simulink model "aircraft_fixd"  (R2016a)
settings: Solver=ode45  StartTime=0.0  StopTime=1000  RelTol=1e-3
undefined symbols (not defined in the file): Newton, Raphson
libraries: simulink x7, aerolibasang x5, aerolib6dof2 x1
settings Model: Creator=HELLO  LastModifiedBy=lsr
settings DataIOCC: LimitDataPoints=on  SaveFormat=Array
settings DebuggingCC: SolverPrmCheckMsg=warning
settings HardwareCC: ProdBitPerPointer=32  ProdLargestAtomicFloat=None  ProdIntDivRoundTo=Undefined  ProdEndianess=Unspecified  ProdWordSize=32  ProdHWDeviceType=32-bit Generic
settings ModelReferenceCC: PropagateSignalLabelsOutOfModel=off
settings ConfigComp: CovModelRefEnable=Off  CovSFcnEnable=off

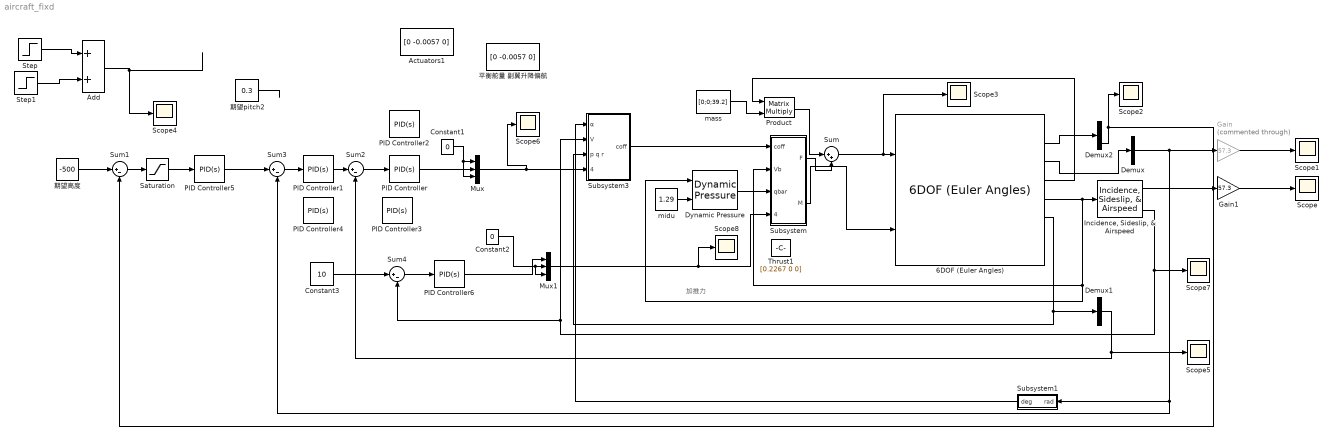
== system aircraft_fixd ==
  note: 加推力
  6DOF (Euler Angles) : aerolib6dof2/6DOF (Euler Angles)  units=Metric (MKS)  mtype=Fixed  rep=Euler Angles  xme_0=[100 0 -200]  Vm_0=[15 0 0]  eul_0=[0 0 0]  pm_0=[0 0 0]  mass_0=4  mass_e=0.5  mass_f=2.0  inertia=[0.1 0 0;0 0.05 0;0 0 0.1]  inertia_e=eye(3)  inertia_f=2*eye(3)  k_quat=1.0  vre_flag=on
  Actuators1 : Constant  Value=[0 -0.0057 0]
  Add : Sum
  Constant1 : Constant  Value=0
  Constant2 : Constant  Value=0
  Constant3 : Constant  Value=10
  Demux : Demux  Outputs=3
  Demux1 : Demux  Outputs=3
  Demux2 : Demux  Outputs=3
  Dynamic Pressure : aerolibasang/Dynamic Pressure
  Gain : Gain  Commented=through  Gain=57.3
  Gain1 : Gain  Gain=57.3
  "Incidence, Sideslip, & Airspeed" : aerolibasang/Incidence, Sideslip, & Airspeed
  Mux : Mux  Inputs=3
  Mux1 : Mux  Inputs=3
  PID Controller : simulink/Continuous/PID Controller  Controller=PID  TimeDomain=Continuous-time  SampleTime=-1  IntegratorMethod=Forward Euler  FilterMethod=Forward Euler  Form=Parallel  UseFilter=on  ControllerParametersSource=internal  P=-0.5  I=-0.01  D=0  N=100  InitialConditionSource=internal  InitialConditionForIntegrator=0  InitialConditionForFilter=0  ExternalReset=none  LimitOutput=off  UpperSaturationLimit=inf  LowerSaturationLimit=-inf  LinearizeAsGain=on  AntiWindupMode=none  Kb=1  TrackingMode=off  Kt=1  PParamMin=[]  PParamMax=[]  IParamMin=[]  IParamMax=[]  DParamMin=[]  DParamMax=[]  NParamMin=[]  NParamMax=[]  KbParamMin=[]  KbParamMax=[]  KtParamMin=[]  KtParamMax=[]  POutMin=[]  POutMax=[]  IOutMin=[]  IOutMax=[]  DOutMin=[]  DOutMax=[]  NOutMin=[]  NOutMax=[]  KbOutMin=[]  KbOutMax=[]  KtOutMin=[]  KtOutMax=[]  IntegratorOutMin=[]  IntegratorOutMax=[]  FilterOutMin=[]  FilterOutMax=[]  SumOutMin=[]  SumOutMax=[]  SumI1OutMin=[]  SumI1OutMax=[]  SumI2OutMin=[]  SumI2OutMax=[]  SumI3OutMin=[]  SumI3OutMax=[]  SumDOutMin=[]  SumDOutMax=[]  SaturationOutMin=[]  SaturationOutMax=[]  IntegratorContinuousStateAttributes=''  IntegratorStateMustResolveToSignalObject=off  IntegratorRTWStateStorageClass=Auto  FilterContinuousStateAttributes=''  FilterStateMustResolveToSignalObject=off  FilterRTWStateStorageClass=Auto  DifferentiatorICPrevScaledInput=0  DifferentiatorOutMin=[]  DifferentiatorOutMax=[]
  PID Controller1 : simulink/Continuous/PID Controller  Controller=PID  TimeDomain=Continuous-time  SampleTime=-1  IntegratorMethod=Forward Euler  FilterMethod=Forward Euler  Form=Parallel  UseFilter=on  ControllerParametersSource=internal  P=0.1  I=0.3  D=0.1  N=100  InitialConditionSource=internal  InitialConditionForIntegrator=0  InitialConditionForFilter=0  ExternalReset=none  LimitOutput=off  UpperSaturationLimit=inf  LowerSaturationLimit=-inf  LinearizeAsGain=on  AntiWindupMode=none  Kb=1  TrackingMode=off  Kt=1  PParamMin=[]  PParamMax=[]  IParamMin=[]  IParamMax=[]  DParamMin=[]  DParamMax=[]  NParamMin=[]  NParamMax=[]  KbParamMin=[]  KbParamMax=[]  KtParamMin=[]  KtParamMax=[]  POutMin=[]  POutMax=[]  IOutMin=[]  IOutMax=[]  DOutMin=[]  DOutMax=[]  NOutMin=[]  NOutMax=[]  KbOutMin=[]  KbOutMax=[]  KtOutMin=[]  KtOutMax=[]  IntegratorOutMin=[]  IntegratorOutMax=[]  FilterOutMin=[]  FilterOutMax=[]  SumOutMin=[]  SumOutMax=[]  SumI1OutMin=[]  SumI1OutMax=[]  SumI2OutMin=[]  SumI2OutMax=[]  SumI3OutMin=[]  SumI3OutMax=[]  SumDOutMin=[]  SumDOutMax=[]  SaturationOutMin=[]  SaturationOutMax=[]  IntegratorContinuousStateAttributes=''  IntegratorStateMustResolveToSignalObject=off  IntegratorRTWStateStorageClass=Auto  FilterContinuousStateAttributes=''  FilterStateMustResolveToSignalObject=off  FilterRTWStateStorageClass=Auto  DifferentiatorICPrevScaledInput=0  DifferentiatorOutMin=[]  DifferentiatorOutMax=[]
  PID Controller2 : simulink/Continuous/PID Controller  Controller=PID  TimeDomain=Continuous-time  SampleTime=-1  IntegratorMethod=Forward Euler  FilterMethod=Forward Euler  Form=Parallel  UseFilter=on  ControllerParametersSource=internal  P=-0.6  I=-0.01  D=0  N=100  InitialConditionSource=internal  InitialConditionForIntegrator=0  InitialConditionForFilter=0  ExternalReset=none  LimitOutput=off  UpperSaturationLimit=inf  LowerSaturationLimit=-inf  LinearizeAsGain=on  AntiWindupMode=none  Kb=1  TrackingMode=off  Kt=1  PParamMin=[]  PParamMax=[]  IParamMin=[]  IParamMax=[]  DParamMin=[]  DParamMax=[]  NParamMin=[]  NParamMax=[]  KbParamMin=[]  KbParamMax=[]  KtParamMin=[]  KtParamMax=[]  POutMin=[]  POutMax=[]  IOutMin=[]  IOutMax=[]  DOutMin=[]  DOutMax=[]  NOutMin=[]  NOutMax=[]  KbOutMin=[]  KbOutMax=[]  KtOutMin=[]  KtOutMax=[]  IntegratorOutMin=[]  IntegratorOutMax=[]  FilterOutMin=[]  FilterOutMax=[]  SumOutMin=[]  SumOutMax=[]  SumI1OutMin=[]  SumI1OutMax=[]  SumI2OutMin=[]  SumI2OutMax=[]  SumI3OutMin=[]  SumI3OutMax=[]  SumDOutMin=[]  SumDOutMax=[]  SaturationOutMin=[]  SaturationOutMax=[]  IntegratorContinuousStateAttributes=''  IntegratorStateMustResolveToSignalObject=off  IntegratorRTWStateStorageClass=Auto  FilterContinuousStateAttributes=''  FilterStateMustResolveToSignalObject=off  FilterRTWStateStorageClass=Auto  DifferentiatorICPrevScaledInput=0  DifferentiatorOutMin=[]  DifferentiatorOutMax=[]
  PID Controller3 : simulink/Continuous/PID Controller  Controller=PID  TimeDomain=Continuous-time  SampleTime=-1  IntegratorMethod=Forward Euler  FilterMethod=Forward Euler  Form=Parallel  UseFilter=on  ControllerParametersSource=internal  P=-0.3  I=-0.01  D=0  N=100  InitialConditionSource=internal  InitialConditionForIntegrator=0  InitialConditionForFilter=0  ExternalReset=none  LimitOutput=off  UpperSaturationLimit=inf  LowerSaturationLimit=-inf  LinearizeAsGain=on  AntiWindupMode=none  Kb=1  TrackingMode=off  Kt=1  PParamMin=[]  PParamMax=[]  IParamMin=[]  IParamMax=[]  DParamMin=[]  DParamMax=[]  NParamMin=[]  NParamMax=[]  KbParamMin=[]  KbParamMax=[]  KtParamMin=[]  KtParamMax=[]  POutMin=[]  POutMax=[]  IOutMin=[]  IOutMax=[]  DOutMin=[]  DOutMax=[]  NOutMin=[]  NOutMax=[]  KbOutMin=[]  KbOutMax=[]  KtOutMin=[]  KtOutMax=[]  IntegratorOutMin=[]  IntegratorOutMax=[]  FilterOutMin=[]  FilterOutMax=[]  SumOutMin=[]  SumOutMax=[]  SumI1OutMin=[]  SumI1OutMax=[]  SumI2OutMin=[]  SumI2OutMax=[]  SumI3OutMin=[]  SumI3OutMax=[]  SumDOutMin=[]  SumDOutMax=[]  SaturationOutMin=[]  SaturationOutMax=[]  IntegratorContinuousStateAttributes=''  IntegratorStateMustResolveToSignalObject=off  IntegratorRTWStateStorageClass=Auto  FilterContinuousStateAttributes=''  FilterStateMustResolveToSignalObject=off  FilterRTWStateStorageClass=Auto  DifferentiatorICPrevScaledInput=0  DifferentiatorOutMin=[]  DifferentiatorOutMax=[]
  PID Controller4 : simulink/Continuous/PID Controller  Controller=PID  TimeDomain=Continuous-time  SampleTime=-1  IntegratorMethod=Forward Euler  FilterMethod=Forward Euler  Form=Parallel  UseFilter=on  ControllerParametersSource=internal  P=0.1  I=0.25  D=0.1  N=100  InitialConditionSource=internal  InitialConditionForIntegrator=0  InitialConditionForFilter=0  ExternalReset=none  LimitOutput=off  UpperSaturationLimit=inf  LowerSaturationLimit=-inf  LinearizeAsGain=on  AntiWindupMode=none  Kb=1  TrackingMode=off  Kt=1  PParamMin=[]  PParamMax=[]  IParamMin=[]  IParamMax=[]  DParamMin=[]  DParamMax=[]  NParamMin=[]  NParamMax=[]  KbParamMin=[]  KbParamMax=[]  KtParamMin=[]  KtParamMax=[]  POutMin=[]  POutMax=[]  IOutMin=[]  IOutMax=[]  DOutMin=[]  DOutMax=[]  NOutMin=[]  NOutMax=[]  KbOutMin=[]  KbOutMax=[]  KtOutMin=[]  KtOutMax=[]  IntegratorOutMin=[]  IntegratorOutMax=[]  FilterOutMin=[]  FilterOutMax=[]  SumOutMin=[]  SumOutMax=[]  SumI1OutMin=[]  SumI1OutMax=[]  SumI2OutMin=[]  SumI2OutMax=[]  SumI3OutMin=[]  SumI3OutMax=[]  SumDOutMin=[]  SumDOutMax=[]  SaturationOutMin=[]  SaturationOutMax=[]  IntegratorContinuousStateAttributes=''  IntegratorStateMustResolveToSignalObject=off  IntegratorRTWStateStorageClass=Auto  FilterContinuousStateAttributes=''  FilterStateMustResolveToSignalObject=off  FilterRTWStateStorageClass=Auto  DifferentiatorICPrevScaledInput=0  DifferentiatorOutMin=[]  DifferentiatorOutMax=[]
  PID Controller5 : simulink/Continuous/PID Controller  Controller=PID  TimeDomain=Continuous-time  SampleTime=-1  IntegratorMethod=Forward Euler  FilterMethod=Forward Euler  Form=Parallel  UseFilter=on  ControllerParametersSource=internal  P=-0.1  I=0  D=0  N=100  InitialConditionSource=internal  InitialConditionForIntegrator=0  InitialConditionForFilter=0  ExternalReset=none  LimitOutput=off  UpperSaturationLimit=inf  LowerSaturationLimit=-inf  LinearizeAsGain=on  AntiWindupMode=none  Kb=1  TrackingMode=off  Kt=1  PParamMin=[]  PParamMax=[]  IParamMin=[]  IParamMax=[]  DParamMin=[]  DParamMax=[]  NParamMin=[]  NParamMax=[]  KbParamMin=[]  KbParamMax=[]  KtParamMin=[]  KtParamMax=[]  POutMin=[]  POutMax=[]  IOutMin=[]  IOutMax=[]  DOutMin=[]  DOutMax=[]  NOutMin=[]  NOutMax=[]  KbOutMin=[]  KbOutMax=[]  KtOutMin=[]  KtOutMax=[]  IntegratorOutMin=[]  IntegratorOutMax=[]  FilterOutMin=[]  FilterOutMax=[]  SumOutMin=[]  SumOutMax=[]  SumI1OutMin=[]  SumI1OutMax=[]  SumI2OutMin=[]  SumI2OutMax=[]  SumI3OutMin=[]  SumI3OutMax=[]  SumDOutMin=[]  SumDOutMax=[]  SaturationOutMin=[]  SaturationOutMax=[]  IntegratorContinuousStateAttributes=''  IntegratorStateMustResolveToSignalObject=off  IntegratorRTWStateStorageClass=Auto  FilterContinuousStateAttributes=''  FilterStateMustResolveToSignalObject=off  FilterRTWStateStorageClass=Auto  DifferentiatorICPrevScaledInput=0  DifferentiatorOutMin=[]  DifferentiatorOutMax=[]
  PID Controller6 : simulink/Continuous/PID Controller  Controller=PID  TimeDomain=Continuous-time  SampleTime=-1  IntegratorMethod=Forward Euler  FilterMethod=Forward Euler  Form=Parallel  UseFilter=on  ControllerParametersSource=internal  P=2  I=0  D=0  N=100  InitialConditionSource=internal  InitialConditionForIntegrator=0  InitialConditionForFilter=0  ExternalReset=none  LimitOutput=off  UpperSaturationLimit=inf  LowerSaturationLimit=-inf  LinearizeAsGain=on  AntiWindupMode=none  Kb=1  TrackingMode=off  Kt=1  PParamMin=[]  PParamMax=[]  IParamMin=[]  IParamMax=[]  DParamMin=[]  DParamMax=[]  NParamMin=[]  NParamMax=[]  KbParamMin=[]  KbParamMax=[]  KtParamMin=[]  KtParamMax=[]  POutMin=[]  POutMax=[]  IOutMin=[]  IOutMax=[]  DOutMin=[]  DOutMax=[]  NOutMin=[]  NOutMax=[]  KbOutMin=[]  KbOutMax=[]  KtOutMin=[]  KtOutMax=[]  IntegratorOutMin=[]  IntegratorOutMax=[]  FilterOutMin=[]  FilterOutMax=[]  SumOutMin=[]  SumOutMax=[]  SumI1OutMin=[]  SumI1OutMax=[]  SumI2OutMin=[]  SumI2OutMax=[]  SumI3OutMin=[]  SumI3OutMax=[]  SumDOutMin=[]  SumDOutMax=[]  SaturationOutMin=[]  SaturationOutMax=[]  IntegratorContinuousStateAttributes=''  IntegratorStateMustResolveToSignalObject=off  IntegratorRTWStateStorageClass=Auto  FilterContinuousStateAttributes=''  FilterStateMustResolveToSignalObject=off  FilterRTWStateStorageClass=Auto  DifferentiatorICPrevScaledInput=0  DifferentiatorOutMin=[]  DifferentiatorOutMax=[]
  Product : Product  Multiplication=Matrix(*)
  Saturation : Saturate  UpperLimit=10  LowerLimit=-10
  Scope{,1..8} (9 alike) : Scope
  Step : Step  Time=2  After=0.1  SampleTime=0
  Step1 : Step  Time=2.1  After=-0.1  SampleTime=0
  Subsystem : Subsystem
  Subsystem1 : Subsystem
  Subsystem3 : Subsystem
  Sum : Sum  Inputs=|++
  Sum{1..4} (4 alike) : Sum  Inputs=|+-
  Thrust1 : Constant  Value=[0.2267 0 0]
  mass : Constant  Value=[0;0;39.2]
  midu : Constant  Value=1.29
  平衡舵量 副翼升降偏航 : Constant  Value=[0 -0.0057 0]
  期望pitch2 : Constant  Value=0.3
  期望高度 : Constant  Value=-500
  wires:
  Subsystem3/1(coff) -> Subsystem/1(coff)
  Mux1/1 -> Scope8/1, Subsystem/4(Thurst)
  Subsystem/2(M) -> 6DOF (Euler Angles)/2
  6DOF (Euler Angles)/5 -> Subsystem/2(Vb), Dynamic Pressure/1, "Incidence, Sideslip, & Airspeed"/1
  6DOF (Euler Angles)/6 -> Demux1/1, Subsystem3/3(p q r)
  midu/1 -> Dynamic Pressure/2
  Dynamic Pressure/1 -> Subsystem/3(qbar)
  mass/1 -> Product/2
  6DOF (Euler Angles)/4 -> Product/1
  Product/1 -> Sum/1
  Sum/1 -> Scope3/1, 6DOF (Euler Angles)/1
  Subsystem/1(F) -> Sum/2
  "Incidence, Sideslip, & Airspeed"/3 -> Scope7/1, Sum4/2, Subsystem3/2(V)
  6DOF (Euler Angles)/2 -> Demux2/1
  "Incidence, Sideslip, & Airspeed"/1 -> Gain1/1
  Subsystem1/1(deg) -> Subsystem3/1(α)
  6DOF (Euler Angles)/3 -> Demux/1
  Demux/2 -> Subsystem1/1(rad), Sum3/2, Gain/1
  Step/1 -> Add/1
  Step1/1 -> Add/2
  Add/1 -> Scope4/1
  Demux1/2 -> Scope5/1, Sum2/2
  Sum2/1 -> PID Controller/1
  PID Controller1/1 -> Sum2/1
  Mux/1 -> Scope6/1, Subsystem3/4(Actuators)
  PID Controller/1 -> Mux/2
  Constant1/1 -> Mux/3, Mux/1
  Sum3/1 -> PID Controller1/1
  PID Controller5/1 -> Sum3/1
  Gain/1 -> Scope1/1
  Gain1/1 -> Scope/1
  Sum1/1 -> Saturation/1
  期望高度/1 -> Sum1/1
  Demux2/3 -> Sum1/2, Scope2/1
  期望pitch2/1 -> ?
  Saturation/1 -> PID Controller5/1
  Constant2/1 -> Mux1/2, Mux1/3
  PID Controller6/1 -> Mux1/1
  Sum4/1 -> PID Controller6/1
  Constant3/1 -> Sum4/1

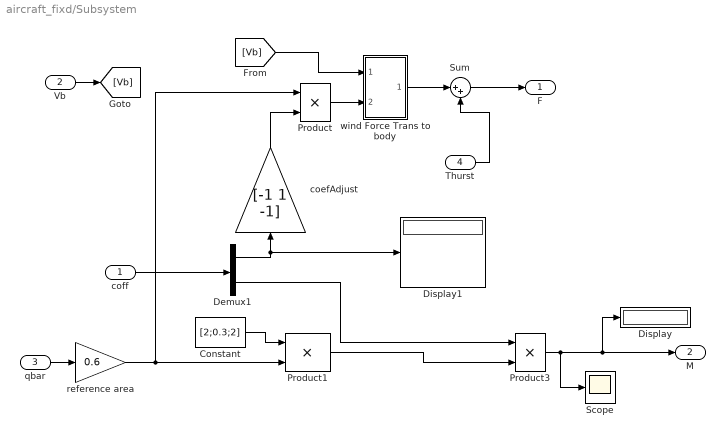
== system aircraft_fixd/Subsystem ==
  coff : Inport
  Vb : Inport  Port=2
  qbar : Inport  Port=3
  Thurst : Inport  Port=4
  Constant : Constant  Value=[2;0.3;2]
  Demux1 : Demux  Outputs=[3,3]
  Display : Display
  Display1 : Display
  Product : Product  SaturateOnIntegerOverflow=on  InputSameDT=on  OutDataTypeStr=Inherit: Same as first input
  Product1 : Product  SaturateOnIntegerOverflow=on  InputSameDT=on  OutDataTypeStr=Inherit: Same as first input
  Product3 : Product  SaturateOnIntegerOverflow=on  InputSameDT=on  OutDataTypeStr=Inherit: Same as first input
  Scope : Scope
  Sum : Sum  Inputs=|++
  coefAdjust : Gain  Gain="[-1  1  -1]"
  reference area : Gain  Gain=0.6  SaturateOnIntegerOverflow=on  OutDataTypeStr=Inherit: Same as input  ParamDataTypeStr=Inherit: Same as input
  wind Force Trans to body : Subsystem
  F : Outport
  M : Outport  Port=2
  wires:
  Product1/1 -> Product3/2
  Constant/1 -> Product1/1
  coff/1 -> Demux1/1
  Demux1/2 -> Product3/1
  qbar/1 -> reference area/1
  reference area/1 -> Product1/2, Product/1
  Demux1/1 -> coefAdjust/1, Display1/1
  Vb/1 -> [Vb]
  coefAdjust/1 -> Product/2
  Thurst/1 -> Sum/2
  Product3/1 -> M/1, Display/1, Scope/1
  Sum/1 -> F/1
  [Vb] -> wind Force Trans to body/1(In1)
  Product/1 -> wind Force Trans to body/2(In2)
  wind Force Trans to body/1(Out1) -> Sum/1

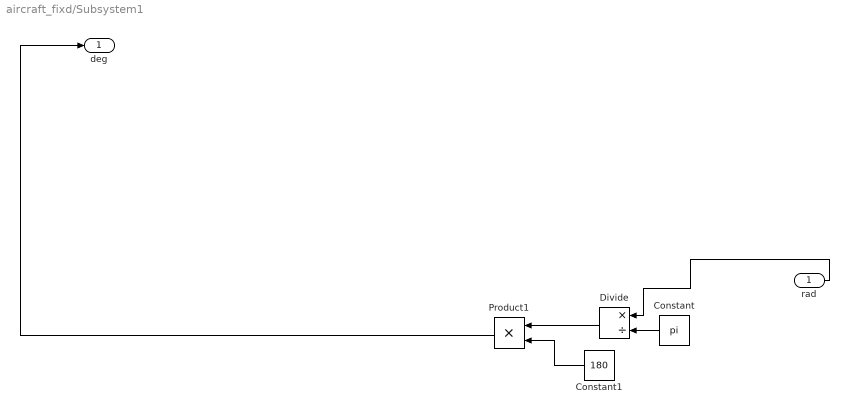
== system aircraft_fixd/Subsystem1 ==
  rad : Inport
  Constant : Constant  Value=pi
  Constant1 : Constant  Value=180
  Divide : Product  Inputs=*/
  Product1 : Product
  deg : Outport
  wires:
  Constant/1 -> Divide/2
  Product1/1 -> deg/1
  Constant1/1 -> Product1/2
  Divide/1 -> Product1/1
  rad/1 -> Divide/1

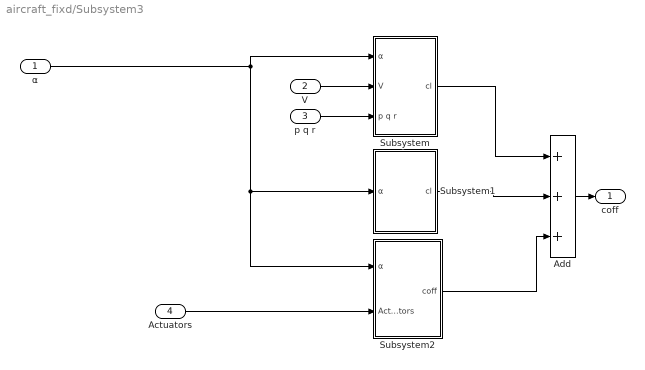
== system aircraft_fixd/Subsystem3 ==
  α : Inport
  V : Inport  Port=2
  p q r : Inport  Port=3
  Actuators : Inport  Port=4
  Add : Sum  Inputs=+++
  Subsystem : Subsystem
  Subsystem1 : Subsystem
  Subsystem2 : Subsystem
  coff : Outport
  wires:
  p q r/1 -> Subsystem/3(p q r)
  V/1 -> Subsystem/2(V)
  Actuators/1 -> Subsystem2/2(Actuators)
  Subsystem1/1(cl) -> Add/2
  Subsystem/1(cl) -> Add/1
  Subsystem2/1(coff) -> Add/3
  Add/1 -> coff/1
  α/1 -> Subsystem/1(α), Subsystem2/1(α), Subsystem1/1(α)

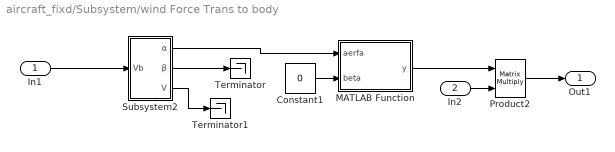
== system aircraft_fixd/Subsystem/wind Force Trans to body ==
  In1 : Inport
  In2 : Inport  Port=2
  Constant1 : Constant  Value=0
  MATLAB Function : MATLAB Function  TreatAsAtomicUnit=on
  Product2 : Product  Multiplication=Matrix(*)  SaturateOnIntegerOverflow=on  InputSameDT=on  OutDataTypeStr=Inherit: Same as first input
  Subsystem2 : Subsystem
  Terminator : Terminator
  Terminator1 : Terminator
  Out1 : Outport
  wires:
  In2/1 -> Product2/2
  In1/1 -> Subsystem2/1(Vb)
  Product2/1 -> Out1/1
  Subsystem2/2(β) -> Terminator/1
  Subsystem2/3(V) -> Terminator1/1
  Subsystem2/1(α) -> MATLAB Function/1(aerfa)
  MATLAB Function/1(y) -> Product2/1
  Constant1/1 -> MATLAB Function/2(beta)

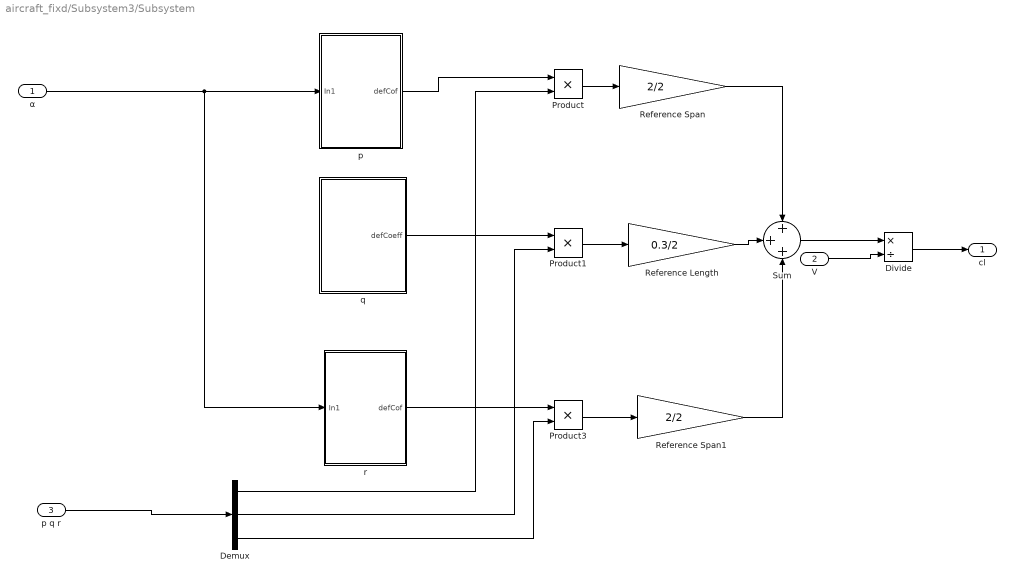
== system aircraft_fixd/Subsystem3/Subsystem ==
  α : Inport
  V : Inport  Port=2
  p q r : Inport  Port=3
  Demux : Demux  Outputs=3
  Divide : Product  Inputs=*/
  Product : Product
  Product1 : Product
  Product3 : Product
  Reference Length : Gain  Gain=0.3/2
  Reference Span : Gain  Gain=2/2
  Reference Span1 : Gain  Gain=2/2
  Sum : Sum  Inputs=+++
  p : Subsystem
  q : Subsystem
  r : Subsystem
  cl : Outport
  wires:
  q/1(defCoeff) -> Product1/1
  p q r/1 -> Demux/1
  p/1(defCof) -> Product/1
  Demux/1 -> Product/2
  Demux/2 -> Product1/2
  r/1(defCof) -> Product3/1
  Demux/3 -> Product3/2
  Product/1 -> Reference Span/1
  Product3/1 -> Reference Span1/1
  Product1/1 -> Reference Length/1
  Reference Span/1 -> Sum/1
  Reference Length/1 -> Sum/2
  Reference Span1/1 -> Sum/3
  Sum/1 -> Divide/1
  V/1 -> Divide/2
  Divide/1 -> cl/1
  α/1 -> r/1(In1), p/1(In1)

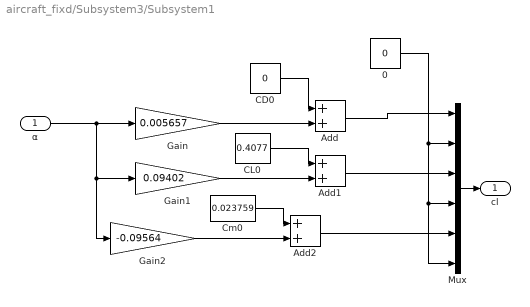
== system aircraft_fixd/Subsystem3/Subsystem1 ==
  α : Inport
  0 : Constant  Value=0
  Add : Sum
  Add1 : Sum
  Add2 : Sum
  CD0 : Constant  Value=0
  CL0 : Constant  Value=0.4077
  Cm0 : Constant  Value=0.023759
  Gain : Gain  Gain=0.005657
  Gain1 : Gain  Gain=0.09402
  Gain2 : Gain  Gain=-0.09564
  Mux : Mux  Inputs=6
  cl : Outport
  wires:
  CD0/1 -> Add/1
  Add/1 -> Mux/1
  Gain1/1 -> Add1/2
  0/1 -> Mux/2, Mux/4, Mux/6
  Add1/1 -> Mux/3
  Gain/1 -> Add/2
  Add2/1 -> Mux/5
  CL0/1 -> Add1/1
  α/1 -> Gain1/1, Gain2/1, Gain/1
  Cm0/1 -> Add2/1
  Gain2/1 -> Add2/2
  Mux/1 -> cl/1

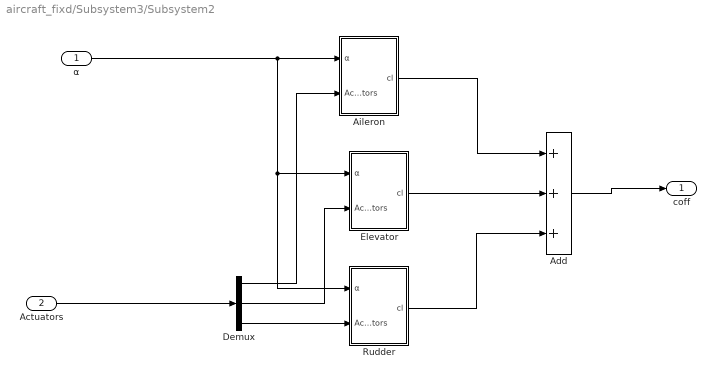
== system aircraft_fixd/Subsystem3/Subsystem2 ==
  α : Inport
  Actuators : Inport  Port=2
  Add : Sum  Inputs=+++
  Aileron : Subsystem
  Demux : Demux  Outputs=3
  Elevator : Subsystem
  Rudder : Subsystem
  coff : Outport
  wires:
  Aileron/1(cl) -> Add/1
  α/1 -> Rudder/1(α), Elevator/1(α), Aileron/1(α)
  Demux/1 -> Aileron/2(Actuators)
  Actuators/1 -> Demux/1
  Rudder/1(cl) -> Add/3
  Elevator/1(cl) -> Add/2
  Demux/3 -> Rudder/2(Actuators)
  Demux/2 -> Elevator/2(Actuators)
  Add/1 -> coff/1

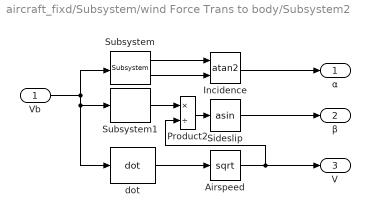
== system aircraft_fixd/Subsystem/wind Force Trans to body/Subsystem2 ==
  Vb : Inport
  Airspeed : Sqrt  AlgorithmType=Newton-Raphson  SaturateOnIntegerOverflow=on
  Incidence : Trigonometry  Operator=atan2
  Product2 : Product  Inputs=*/  SaturateOnIntegerOverflow=on  OutDataTypeStr=Inherit: Same as first input
  Sideslip : Trigonometry  Operator=asin
  Subsystem : aerolibasang/Incidence, Sideslip, & Airspeed/Subsystem
  Subsystem1 : aerolibasang/Incidence, Sideslip, & Airspeed/Subsystem1
  dot : aerolibasang/Incidence, Sideslip, & Airspeed/dot
  α : Outport
  β : Outport  Port=2
  V : Outport  Port=3
  wires:
  Subsystem1/1 -> Product2/1
  Sideslip/1 -> β/1
  Vb/1 -> Subsystem/1, dot/1, Subsystem1/1
  Incidence/1 -> α/1
  Airspeed/1 -> V/1, Product2/2
  dot/1 -> Airspeed/1
  Subsystem/2 -> Incidence/2
  Subsystem/1 -> Incidence/1
  Product2/1 -> Sideslip/1

== system aircraft_fixd/Subsystem3/Subsystem/p ==
  In1 : Inport
  Constant : Constant  Value=0
  Mux : Mux  Inputs=6
  defCof : Outport
  wires:
  Mux/1 -> defCof/1
  Constant/1 -> Mux/1, Mux/2, Mux/3, Mux/4, Mux/5, Mux/6

== system aircraft_fixd/Subsystem3/Subsystem/q ==
  CmQ1 : Constant  Value=-5
  CmQ3 : Constant  Value=-63.8
  Constant : Constant  Value=0
  Mux : Mux  Inputs=6
  defCoeff : Outport
  wires:
  CmQ1/1 -> Mux/5
  Mux/1 -> defCoeff/1
  Constant/1 -> Mux/1, Mux/2, Mux/3, Mux/4, Mux/6

== system aircraft_fixd/Subsystem3/Subsystem/r ==
  In1 : Inport
  Constant : Constant  Value=0
  Mux : Mux  Inputs=6
  defCof : Outport
  wires:
  Mux/1 -> defCof/1
  Constant/1 -> Mux/1, Mux/2, Mux/3, Mux/4, Mux/5, Mux/6

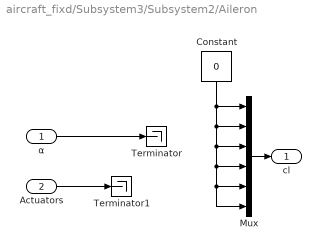
== system aircraft_fixd/Subsystem3/Subsystem2/Aileron ==
  α : Inport
  Actuators : Inport  Port=2
  Constant : Constant  Value=0
  Mux : Mux  Inputs=6
  Terminator : Terminator
  Terminator1 : Terminator
  cl : Outport
  wires:
  Constant/1 -> Mux/1, Mux/2, Mux/3, Mux/4, Mux/5, Mux/6
  α/1 -> Terminator/1
  Mux/1 -> cl/1
  Actuators/1 -> Terminator1/1

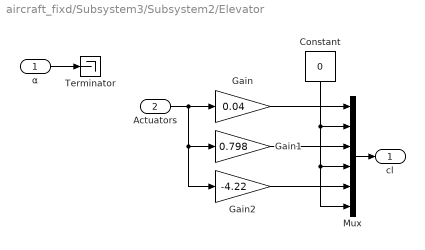
== system aircraft_fixd/Subsystem3/Subsystem2/Elevator ==
  α : Inport
  Actuators : Inport  Port=2
  Constant : Constant  Value=0
  Gain : Gain  Gain=0.04
  Gain1 : Gain  Gain=0.798
  Gain2 : Gain  Gain=-4.22
  Mux : Mux  Inputs=6
  Terminator : Terminator
  cl : Outport
  wires:
  Actuators/1 -> Gain2/1, Gain1/1, Gain/1
  Mux/1 -> cl/1
  α/1 -> Terminator/1
  Constant/1 -> Mux/6, Mux/4, Mux/2
  Gain/1 -> Mux/1
  Gain1/1 -> Mux/3
  Gain2/1 -> Mux/5

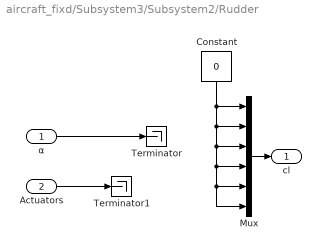
== system aircraft_fixd/Subsystem3/Subsystem2/Rudder ==
  α : Inport
  Actuators : Inport  Port=2
  Constant : Constant  Value=0
  Mux : Mux  Inputs=6
  Terminator : Terminator
  Terminator1 : Terminator
  cl : Outport
  wires:
  Constant/1 -> Mux/1, Mux/2, Mux/3, Mux/4, Mux/5, Mux/6
  α/1 -> Terminator/1
  Mux/1 -> cl/1
  Actuators/1 -> Terminator1/1

== matlab function aircraft_fixd/Subsystem/wind Force Trans to body/MATLAB Function ==
  data: aerfa input; y output; beta input
function y = fcn(aerfa,beta)   %输入为倾角beta，和迎角aerfa    %风轴系到体轴系的变换矩阵



a = cos(aerfa)*cos(beta);
b = -cos(aerfa)*sin(beta);
c = -sin(aerfa);

d = sin(beta);
e = cos(beta);
f = 0;

g = sin(aerfa)*cos(beta);
h = -sin(beta)*sin(aerfa);
i = cos(aerfa);



y = [a,b,c;d,e,f;g,h,i];
